simulink model "CM475A_TSG31CfgAndUse"  (R2013b)
settings: Solver=FixedStepDiscrete  SolverMode=SingleTasking  StartTime=0.0  StopTime=0.5  FixedStep=0.00005  RelTol=1e-3
undefined symbols (not defined in the file): ELECGLBPRM_PWMPERDMIN_NANOSEC_U32, sigbuilder_block, SysSt1, TSG31CfgAndUseAdcStrtOfCnvn2Offs, TSG31CfgAndUseAdcStrtOfCnvnMotCtrlPeakOffs, TSG31CfgAndUseAdcStrtOfCnvnMotCtrlVlyOffs, TSG31CfgAndUseMtrAg0SPIStart, TSG31CfgAndUsePwmDbnd, TSG31UPD_NANOSEC_U32
libraries: simulink x11, CM475A_TSG31CfgAndUse_ModelLibrary_Rev001 x11
(part 2 of 4)

== system CM475A_TSG31CfgAndUse/TSG31CfgAndUse/TSG31CfgAndUsePer2/No Transition SysState = Enable/MCECS_GAINCMDCF ==
  Action Port : ActionPort  ActionType=case
  CopyRight2 : Subsystem  Description=|  mask(Copyright Information){none=on}
      | Copyright info block.                                               
      |                                                                     
      | Place copyright information at the top of every subsystem in design.
      mask prompts: none "No parameters"
      mask help: Place copyright information at the top of every subsystem in design.
      mask Display:
      | NxtrConf = 'Nexteer Confidential';
      | 
      | sys = bdroot; %handle for the current model ("system")
      | first = get_param(sys,'Created');
      | first = first(end-3:end);  %year is last four digits
      | 
      | last = get_param(sys,'LastModifiedDate');
      | if isempty(last)
      |     last = datestr(now,'yyyy');
      | else
      |     last = last(end-3:end);
      | end
      | 
      | if strcmp(first,last)
      |     fprintf('%s -- Copyright %s Nexteer',NxtrConf,first)
      | else
      |     fprintf('%s -- %s%s- %s Nexteer',NxtrConf,char(169),first,last)
      | end
  Map Pins to GPIO : Subsystem  Priority=10  TreatAsAtomicUnit=on
      settings: AttributesFormatString=|
      | Priority:
      | %<Priority>
  Set GPIO Level : Subsystem  Priority=20  TreatAsAtomicUnit=on
      settings: AttributesFormatString=|
      | Priority:
      | %<Priority>

== system CM475A_TSG31CfgAndUse/TSG31CfgAndUse/TSG31CfgAndUsePer2/No Transition SysState = Enable/MCECS_OFFSCMDEND and MCECS_GAINCMDAD ==
  Action Port : ActionPort  ActionType=case
  CopyRight2 : Subsystem  Description=|  mask(Copyright Information){none=on}
      | Copyright info block.                                               
      |                                                                     
      | Place copyright information at the top of every subsystem in design.
      mask prompts: none "No parameters"
      mask help: Place copyright information at the top of every subsystem in design.
      mask Display:
      | NxtrConf = 'Nexteer Confidential';
      | 
      | sys = bdroot; %handle for the current model ("system")
      | first = get_param(sys,'Created');
      | first = first(end-3:end);  %year is last four digits
      | 
      | last = get_param(sys,'LastModifiedDate');
      | if isempty(last)
      |     last = datestr(now,'yyyy');
      | else
      |     last = last(end-3:end);
      | end
      | 
      | if strcmp(first,last)
      |     fprintf('%s -- Copyright %s Nexteer',NxtrConf,first)
      | else
      |     fprintf('%s -- %s%s- %s Nexteer',NxtrConf,char(169),first,last)
      | end
  Map Pins to GPIO : Subsystem  Priority=10  TreatAsAtomicUnit=on
      settings: AttributesFormatString=|
      | Priority:
      | %<Priority>
  Set GPIO Level : Subsystem  Priority=20  TreatAsAtomicUnit=on
      settings: AttributesFormatString=|
      | Priority:
      | %<Priority>

== system CM475A_TSG31CfgAndUse/TSG31CfgAndUse/TSG31CfgAndUsePer2/Transition from Enable/CopyRight2 ==

== system CM475A_TSG31CfgAndUse/TSG31CfgAndUse/TSG31CfgAndUsePer2/Transition from Enable/Map FET Ctrl Signals to GPIO and Set Low ==
  CopyRight2 : Subsystem  Description=|  mask(Copyright Information){none=on}
      | Copyright info block.                                               
      |                                                                     
      | Place copyright information at the top of every subsystem in design.
      mask prompts: none "No parameters"
      mask help: Place copyright information at the top of every subsystem in design.
      mask Display:
      | NxtrConf = 'Nexteer Confidential';
      | 
      | sys = bdroot; %handle for the current model ("system")
      | first = get_param(sys,'Created');
      | first = first(end-3:end);  %year is last four digits
      | 
      | last = get_param(sys,'LastModifiedDate');
      | if isempty(last)
      |     last = datestr(now,'yyyy');
      | else
      |     last = last(end-3:end);
      | end
      | 
      | if strcmp(first,last)
      |     fprintf('%s -- Copyright %s Nexteer',NxtrConf,first)
      | else
      |     fprintf('%s -- %s%s- %s Nexteer',NxtrConf,char(169),first,last)
      | end
  Map Pins to GPIO : Subsystem  RequirementInfo={'linktype_rmi_doors' '000089b8 (/ESG Group/FDD Module Requirements/ES FDDs/CM475A - TSG31 Configuration and Use)' '#CM475A_15' 'true' 'REQ: CM475A_15' '' } %GIDa_06ec1fec_3e1a_4ad4_824a_b175bdae6a2a  Priority=10  TreatAsAtomicUnit=on
      settings: AttributesFormatString=|
      | Priority:
      | %<Priority>
  Set GPIO Level : Subsystem  Priority=20  TreatAsAtomicUnit=on
      settings: AttributesFormatString=|
      | Priority:
      | %<Priority>

== system CM475A_TSG31CfgAndUse/TSG31CfgAndUse/TSG31CfgAndUsePer2/Transition to Enable/CopyRight2 ==

== system CM475A_TSG31CfgAndUse/TSG31CfgAndUse/TSG31CfgAndUsePer2/Transition to Enable/Map Pins to Peripheral ==
  IoHwAb_SetFctPeriphPhaALowrCmd : Subsystem  TreatAsAtomicUnit=on
  IoHwAb_SetFctPeriphPhaAUpprCmd : Subsystem  TreatAsAtomicUnit=on
  IoHwAb_SetFctPeriphPhaBLowrCmd : Subsystem  TreatAsAtomicUnit=on
  IoHwAb_SetFctPeriphPhaBUpprCmd : Subsystem  TreatAsAtomicUnit=on
  IoHwAb_SetFctPeriphPhaCLowrCmd : Subsystem  TreatAsAtomicUnit=on
  IoHwAb_SetFctPeriphPhaCUpprCmd : Subsystem  TreatAsAtomicUnit=on

== system CM475A_TSG31CfgAndUse/TSG31CfgAndUse/TSG31CfgAndUseInit1/Map FET Ctrl Signals to GPIO and Set Low/Map Pins to GPIO/CopyRight2 ==

== system CM475A_TSG31CfgAndUse/TSG31CfgAndUse/TSG31CfgAndUseInit1/Map FET Ctrl Signals to GPIO and Set Low/Map Pins to GPIO/IoHwAb_SetFctGpioPhaALowrCmd ==
  CopyRight2 : Subsystem  Description=|  mask(Copyright Information){none=on}
      | Copyright info block.                                               
      |                                                                     
      | Place copyright information at the top of every subsystem in design.
      mask prompts: none "No parameters"
      mask help: Place copyright information at the top of every subsystem in design.
      mask Display:
      | NxtrConf = 'Nexteer Confidential';
      | 
      | sys = bdroot; %handle for the current model ("system")
      | first = get_param(sys,'Created');
      | first = first(end-3:end);  %year is last four digits
      | 
      | last = get_param(sys,'LastModifiedDate');
      | if isempty(last)
      |     last = datestr(now,'yyyy');
      | else
      |     last = last(end-3:end);
      | end
      | 
      | if strcmp(first,last)
      |     fprintf('%s -- Copyright %s Nexteer',NxtrConf,first)
      | else
      |     fprintf('%s -- %s%s- %s Nexteer',NxtrConf,char(169),first,last)
      | end

== system CM475A_TSG31CfgAndUse/TSG31CfgAndUse/TSG31CfgAndUseInit1/Map FET Ctrl Signals to GPIO and Set Low/Map Pins to GPIO/IoHwAb_SetFctGpioPhaAUpprCmd ==
  CopyRight2 : Subsystem  Description=|  mask(Copyright Information){none=on}
      | Copyright info block.                                               
      |                                                                     
      | Place copyright information at the top of every subsystem in design.
      mask prompts: none "No parameters"
      mask help: Place copyright information at the top of every subsystem in design.
      mask Display:
      | NxtrConf = 'Nexteer Confidential';
      | 
      | sys = bdroot; %handle for the current model ("system")
      | first = get_param(sys,'Created');
      | first = first(end-3:end);  %year is last four digits
      | 
      | last = get_param(sys,'LastModifiedDate');
      | if isempty(last)
      |     last = datestr(now,'yyyy');
      | else
      |     last = last(end-3:end);
      | end
      | 
      | if strcmp(first,last)
      |     fprintf('%s -- Copyright %s Nexteer',NxtrConf,first)
      | else
      |     fprintf('%s -- %s%s- %s Nexteer',NxtrConf,char(169),first,last)
      | end

== system CM475A_TSG31CfgAndUse/TSG31CfgAndUse/TSG31CfgAndUseInit1/Map FET Ctrl Signals to GPIO and Set Low/Map Pins to GPIO/IoHwAb_SetFctGpioPhaBLowrCmd ==
  CopyRight2 : Subsystem  Description=|  mask(Copyright Information){none=on}
      | Copyright info block.                                               
      |                                                                     
      | Place copyright information at the top of every subsystem in design.
      mask prompts: none "No parameters"
      mask help: Place copyright information at the top of every subsystem in design.
      mask Display:
      | NxtrConf = 'Nexteer Confidential';
      | 
      | sys = bdroot; %handle for the current model ("system")
      | first = get_param(sys,'Created');
      | first = first(end-3:end);  %year is last four digits
      | 
      | last = get_param(sys,'LastModifiedDate');
      | if isempty(last)
      |     last = datestr(now,'yyyy');
      | else
      |     last = last(end-3:end);
      | end
      | 
      | if strcmp(first,last)
      |     fprintf('%s -- Copyright %s Nexteer',NxtrConf,first)
      | else
      |     fprintf('%s -- %s%s- %s Nexteer',NxtrConf,char(169),first,last)
      | end

== system CM475A_TSG31CfgAndUse/TSG31CfgAndUse/TSG31CfgAndUseInit1/Map FET Ctrl Signals to GPIO and Set Low/Map Pins to GPIO/IoHwAb_SetFctGpioPhaBUpprCmd ==
  CopyRight2 : Subsystem  Description=|  mask(Copyright Information){none=on}
      | Copyright info block.                                               
      |                                                                     
      | Place copyright information at the top of every subsystem in design.
      mask prompts: none "No parameters"
      mask help: Place copyright information at the top of every subsystem in design.
      mask Display:
      | NxtrConf = 'Nexteer Confidential';
      | 
      | sys = bdroot; %handle for the current model ("system")
      | first = get_param(sys,'Created');
      | first = first(end-3:end);  %year is last four digits
      | 
      | last = get_param(sys,'LastModifiedDate');
      | if isempty(last)
      |     last = datestr(now,'yyyy');
      | else
      |     last = last(end-3:end);
      | end
      | 
      | if strcmp(first,last)
      |     fprintf('%s -- Copyright %s Nexteer',NxtrConf,first)
      | else
      |     fprintf('%s -- %s%s- %s Nexteer',NxtrConf,char(169),first,last)
      | end

== system CM475A_TSG31CfgAndUse/TSG31CfgAndUse/TSG31CfgAndUseInit1/Map FET Ctrl Signals to GPIO and Set Low/Map Pins to GPIO/IoHwAb_SetFctGpioPhaCLowrCmd ==
  CopyRight2 : Subsystem  Description=|  mask(Copyright Information){none=on}
      | Copyright info block.                                               
      |                                                                     
      | Place copyright information at the top of every subsystem in design.
      mask prompts: none "No parameters"
      mask help: Place copyright information at the top of every subsystem in design.
      mask Display:
      | NxtrConf = 'Nexteer Confidential';
      | 
      | sys = bdroot; %handle for the current model ("system")
      | first = get_param(sys,'Created');
      | first = first(end-3:end);  %year is last four digits
      | 
      | last = get_param(sys,'LastModifiedDate');
      | if isempty(last)
      |     last = datestr(now,'yyyy');
      | else
      |     last = last(end-3:end);
      | end
      | 
      | if strcmp(first,last)
      |     fprintf('%s -- Copyright %s Nexteer',NxtrConf,first)
      | else
      |     fprintf('%s -- %s%s- %s Nexteer',NxtrConf,char(169),first,last)
      | end

== system CM475A_TSG31CfgAndUse/TSG31CfgAndUse/TSG31CfgAndUseInit1/Map FET Ctrl Signals to GPIO and Set Low/Map Pins to GPIO/IoHwAb_SetFctGpioPhaCUpprCmd ==
  CopyRight2 : Subsystem  Description=|  mask(Copyright Information){none=on}
      | Copyright info block.                                               
      |                                                                     
      | Place copyright information at the top of every subsystem in design.
      mask prompts: none "No parameters"
      mask help: Place copyright information at the top of every subsystem in design.
      mask Display:
      | NxtrConf = 'Nexteer Confidential';
      | 
      | sys = bdroot; %handle for the current model ("system")
      | first = get_param(sys,'Created');
      | first = first(end-3:end);  %year is last four digits
      | 
      | last = get_param(sys,'LastModifiedDate');
      | if isempty(last)
      |     last = datestr(now,'yyyy');
      | else
      |     last = last(end-3:end);
      | end
      | 
      | if strcmp(first,last)
      |     fprintf('%s -- Copyright %s Nexteer',NxtrConf,first)
      | else
      |     fprintf('%s -- %s%s- %s Nexteer',NxtrConf,char(169),first,last)
      | end

== system CM475A_TSG31CfgAndUse/TSG31CfgAndUse/TSG31CfgAndUseInit1/Map FET Ctrl Signals to GPIO and Set Low/Set GPIO Level/CopyRight2 ==

== system CM475A_TSG31CfgAndUse/TSG31CfgAndUse/TSG31CfgAndUseInit1/Map FET Ctrl Signals to GPIO and Set Low/Set GPIO Level/IoHwAb_SetGpioPhaALowrCmd ==
  PinSt : Inport  OutDataTypeStr=boolean
  CopyRight2 : Subsystem  Description=|  mask(Copyright Information){none=on}
      | Copyright info block.                                               
      |                                                                     
      | Place copyright information at the top of every subsystem in design.
      mask prompts: none "No parameters"
      mask help: Place copyright information at the top of every subsystem in design.
      mask Display:
      | NxtrConf = 'Nexteer Confidential';
      | 
      | sys = bdroot; %handle for the current model ("system")
      | first = get_param(sys,'Created');
      | first = first(end-3:end);  %year is last four digits
      | 
      | last = get_param(sys,'LastModifiedDate');
      | if isempty(last)
      |     last = datestr(now,'yyyy');
      | else
      |     last = last(end-3:end);
      | end
      | 
      | if strcmp(first,last)
      |     fprintf('%s -- Copyright %s Nexteer',NxtrConf,first)
      | else
      |     fprintf('%s -- %s%s- %s Nexteer',NxtrConf,char(169),first,last)
      | end
  Terminator : Terminator
  wires:
  PinSt/1 -> Terminator/1

== system CM475A_TSG31CfgAndUse/TSG31CfgAndUse/TSG31CfgAndUseInit1/Map FET Ctrl Signals to GPIO and Set Low/Set GPIO Level/IoHwAb_SetGpioPhaAUpprCmd ==
  PinSt : Inport  OutDataTypeStr=boolean
  CopyRight2 : Subsystem  Description=|  mask(Copyright Information){none=on}
      | Copyright info block.                                               
      |                                                                     
      | Place copyright information at the top of every subsystem in design.
      mask prompts: none "No parameters"
      mask help: Place copyright information at the top of every subsystem in design.
      mask Display:
      | NxtrConf = 'Nexteer Confidential';
      | 
      | sys = bdroot; %handle for the current model ("system")
      | first = get_param(sys,'Created');
      | first = first(end-3:end);  %year is last four digits
      | 
      | last = get_param(sys,'LastModifiedDate');
      | if isempty(last)
      |     last = datestr(now,'yyyy');
      | else
      |     last = last(end-3:end);
      | end
      | 
      | if strcmp(first,last)
      |     fprintf('%s -- Copyright %s Nexteer',NxtrConf,first)
      | else
      |     fprintf('%s -- %s%s- %s Nexteer',NxtrConf,char(169),first,last)
      | end
  Terminator : Terminator
  wires:
  PinSt/1 -> Terminator/1

== system CM475A_TSG31CfgAndUse/TSG31CfgAndUse/TSG31CfgAndUseInit1/Map FET Ctrl Signals to GPIO and Set Low/Set GPIO Level/IoHwAb_SetGpioPhaBLowrCmd ==
  PinSt : Inport  OutDataTypeStr=boolean
  CopyRight2 : Subsystem  Description=|  mask(Copyright Information){none=on}
      | Copyright info block.                                               
      |                                                                     
      | Place copyright information at the top of every subsystem in design.
      mask prompts: none "No parameters"
      mask help: Place copyright information at the top of every subsystem in design.
      mask Display:
      | NxtrConf = 'Nexteer Confidential';
      | 
      | sys = bdroot; %handle for the current model ("system")
      | first = get_param(sys,'Created');
      | first = first(end-3:end);  %year is last four digits
      | 
      | last = get_param(sys,'LastModifiedDate');
      | if isempty(last)
      |     last = datestr(now,'yyyy');
      | else
      |     last = last(end-3:end);
      | end
      | 
      | if strcmp(first,last)
      |     fprintf('%s -- Copyright %s Nexteer',NxtrConf,first)
      | else
      |     fprintf('%s -- %s%s- %s Nexteer',NxtrConf,char(169),first,last)
      | end
  Terminator : Terminator
  wires:
  PinSt/1 -> Terminator/1

== system CM475A_TSG31CfgAndUse/TSG31CfgAndUse/TSG31CfgAndUseInit1/Map FET Ctrl Signals to GPIO and Set Low/Set GPIO Level/IoHwAb_SetGpioPhaBUpprCmd ==
  PinSt : Inport  OutDataTypeStr=boolean
  CopyRight2 : Subsystem  Description=|  mask(Copyright Information){none=on}
      | Copyright info block.                                               
      |                                                                     
      | Place copyright information at the top of every subsystem in design.
      mask prompts: none "No parameters"
      mask help: Place copyright information at the top of every subsystem in design.
      mask Display:
      | NxtrConf = 'Nexteer Confidential';
      | 
      | sys = bdroot; %handle for the current model ("system")
      | first = get_param(sys,'Created');
      | first = first(end-3:end);  %year is last four digits
      | 
      | last = get_param(sys,'LastModifiedDate');
      | if isempty(last)
      |     last = datestr(now,'yyyy');
      | else
      |     last = last(end-3:end);
      | end
      | 
      | if strcmp(first,last)
      |     fprintf('%s -- Copyright %s Nexteer',NxtrConf,first)
      | else
      |     fprintf('%s -- %s%s- %s Nexteer',NxtrConf,char(169),first,last)
      | end
  Terminator : Terminator
  wires:
  PinSt/1 -> Terminator/1

== system CM475A_TSG31CfgAndUse/TSG31CfgAndUse/TSG31CfgAndUseInit1/Map FET Ctrl Signals to GPIO and Set Low/Set GPIO Level/IoHwAb_SetGpioPhaCLowrCmd ==
  PinSt : Inport  OutDataTypeStr=boolean
  CopyRight2 : Subsystem  Description=|  mask(Copyright Information){none=on}
      | Copyright info block.                                               
      |                                                                     
      | Place copyright information at the top of every subsystem in design.
      mask prompts: none "No parameters"
      mask help: Place copyright information at the top of every subsystem in design.
      mask Display:
      | NxtrConf = 'Nexteer Confidential';
      | 
      | sys = bdroot; %handle for the current model ("system")
      | first = get_param(sys,'Created');
      | first = first(end-3:end);  %year is last four digits
      | 
      | last = get_param(sys,'LastModifiedDate');
      | if isempty(last)
      |     last = datestr(now,'yyyy');
      | else
      |     last = last(end-3:end);
      | end
      | 
      | if strcmp(first,last)
      |     fprintf('%s -- Copyright %s Nexteer',NxtrConf,first)
      | else
      |     fprintf('%s -- %s%s- %s Nexteer',NxtrConf,char(169),first,last)
      | end
  Terminator : Terminator
  wires:
  PinSt/1 -> Terminator/1

== system CM475A_TSG31CfgAndUse/TSG31CfgAndUse/TSG31CfgAndUseInit1/Map FET Ctrl Signals to GPIO and Set Low/Set GPIO Level/IoHwAb_SetGpioPhaCUpprCmd ==
  PinSt : Inport  OutDataTypeStr=boolean
  CopyRight2 : Subsystem  Description=|  mask(Copyright Information){none=on}
      | Copyright info block.                                               
      |                                                                     
      | Place copyright information at the top of every subsystem in design.
      mask prompts: none "No parameters"
      mask help: Place copyright information at the top of every subsystem in design.
      mask Display:
      | NxtrConf = 'Nexteer Confidential';
      | 
      | sys = bdroot; %handle for the current model ("system")
      | first = get_param(sys,'Created');
      | first = first(end-3:end);  %year is last four digits
      | 
      | last = get_param(sys,'LastModifiedDate');
      | if isempty(last)
      |     last = datestr(now,'yyyy');
      | else
      |     last = last(end-3:end);
      | end
      | 
      | if strcmp(first,last)
      |     fprintf('%s -- Copyright %s Nexteer',NxtrConf,first)
      | else
      |     fprintf('%s -- %s%s- %s Nexteer',NxtrConf,char(169),first,last)
      | end
  Terminator : Terminator
  wires:
  PinSt/1 -> Terminator/1

== system CM475A_TSG31CfgAndUse/TSG31CfgAndUse/TSG31CfgAndUsePer2/No Transition SysState = Enable/Do Nothing/CopyRight2 ==

== system CM475A_TSG31CfgAndUse/TSG31CfgAndUse/TSG31CfgAndUsePer2/No Transition SysState = Enable/MCECS_CMDSAFEST/CopyRight2 ==

== system CM475A_TSG31CfgAndUse/TSG31CfgAndUse/TSG31CfgAndUsePer2/No Transition SysState = Enable/MCECS_CMDSAFEST/Map Pins to GPIO ==
  CopyRight2 : Subsystem  Description=|  mask(Copyright Information){none=on}
      | Copyright info block.                                               
      |                                                                     
      | Place copyright information at the top of every subsystem in design.
      mask prompts: none "No parameters"
      mask help: Place copyright information at the top of every subsystem in design.
      mask Display:
      | NxtrConf = 'Nexteer Confidential';
      | 
      | sys = bdroot; %handle for the current model ("system")
      | first = get_param(sys,'Created');
      | first = first(end-3:end);  %year is last four digits
      | 
      | last = get_param(sys,'LastModifiedDate');
      | if isempty(last)
      |     last = datestr(now,'yyyy');
      | else
      |     last = last(end-3:end);
      | end
      | 
      | if strcmp(first,last)
      |     fprintf('%s -- Copyright %s Nexteer',NxtrConf,first)
      | else
      |     fprintf('%s -- %s%s- %s Nexteer',NxtrConf,char(169),first,last)
      | end
  IoHwAb_SetFctGpioPhaALowrCmd : Subsystem  TreatAsAtomicUnit=on
  IoHwAb_SetFctGpioPhaAUpprCmd : Subsystem  TreatAsAtomicUnit=on
  IoHwAb_SetFctGpioPhaBLowrCmd : Subsystem  TreatAsAtomicUnit=on
  IoHwAb_SetFctGpioPhaBUpprCmd : Subsystem  TreatAsAtomicUnit=on
  IoHwAb_SetFctGpioPhaCLowrCmd : Subsystem  TreatAsAtomicUnit=on
  IoHwAb_SetFctGpioPhaCUpprCmd : Subsystem  TreatAsAtomicUnit=on

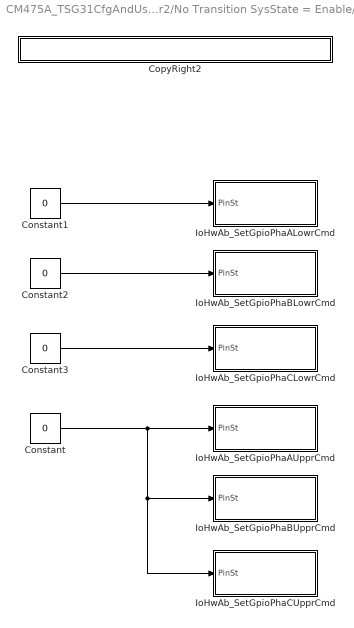
== system CM475A_TSG31CfgAndUse/TSG31CfgAndUse/TSG31CfgAndUsePer2/No Transition SysState = Enable/MCECS_CMDSAFEST/Set GPIO Level ==
  Constant{,1..3} (4 alike) : Constant  Value=0  OutDataTypeStr=boolean
  CopyRight2 : Subsystem  Description=|  mask(Copyright Information){none=on}
      | Copyright info block.                                               
      |                                                                     
      | Place copyright information at the top of every subsystem in design.
      mask prompts: none "No parameters"
      mask help: Place copyright information at the top of every subsystem in design.
      mask Display:
      | NxtrConf = 'Nexteer Confidential';
      | 
      | sys = bdroot; %handle for the current model ("system")
      | first = get_param(sys,'Created');
      | first = first(end-3:end);  %year is last four digits
      | 
      | last = get_param(sys,'LastModifiedDate');
      | if isempty(last)
      |     last = datestr(now,'yyyy');
      | else
      |     last = last(end-3:end);
      | end
      | 
      | if strcmp(first,last)
      |     fprintf('%s -- Copyright %s Nexteer',NxtrConf,first)
      | else
      |     fprintf('%s -- %s%s- %s Nexteer',NxtrConf,char(169),first,last)
      | end
  IoHwAb_SetGpioPhaALowrCmd : Subsystem  TreatAsAtomicUnit=on
  IoHwAb_SetGpioPhaAUpprCmd : Subsystem  TreatAsAtomicUnit=on
  IoHwAb_SetGpioPhaBLowrCmd : Subsystem  TreatAsAtomicUnit=on
  IoHwAb_SetGpioPhaBUpprCmd : Subsystem  TreatAsAtomicUnit=on
  IoHwAb_SetGpioPhaCLowrCmd : Subsystem  TreatAsAtomicUnit=on
  IoHwAb_SetGpioPhaCUpprCmd : Subsystem  TreatAsAtomicUnit=on
  wires:
  Constant3/1 -> IoHwAb_SetGpioPhaCLowrCmd/1(PinSt)
  Constant2/1 -> IoHwAb_SetGpioPhaBLowrCmd/1(PinSt)
  Constant1/1 -> IoHwAb_SetGpioPhaALowrCmd/1(PinSt)
  Constant/1 -> IoHwAb_SetGpioPhaAUpprCmd/1(PinSt), IoHwAb_SetGpioPhaBUpprCmd/1(PinSt), IoHwAb_SetGpioPhaCUpprCmd/1(PinSt)

== system CM475A_TSG31CfgAndUse/TSG31CfgAndUse/TSG31CfgAndUsePer2/No Transition SysState = Enable/MCECS_GAINCMDBE/CopyRight2 ==

== system CM475A_TSG31CfgAndUse/TSG31CfgAndUse/TSG31CfgAndUsePer2/No Transition SysState = Enable/MCECS_GAINCMDBE/Map Pins to GPIO ==
  CopyRight2 : Subsystem  Description=|  mask(Copyright Information){none=on}
      | Copyright info block.                                               
      |                                                                     
      | Place copyright information at the top of every subsystem in design.
      mask prompts: none "No parameters"
      mask help: Place copyright information at the top of every subsystem in design.
      mask Display:
      | NxtrConf = 'Nexteer Confidential';
      | 
      | sys = bdroot; %handle for the current model ("system")
      | first = get_param(sys,'Created');
      | first = first(end-3:end);  %year is last four digits
      | 
      | last = get_param(sys,'LastModifiedDate');
      | if isempty(last)
      |     last = datestr(now,'yyyy');
      | else
      |     last = last(end-3:end);
      | end
      | 
      | if strcmp(first,last)
      |     fprintf('%s -- Copyright %s Nexteer',NxtrConf,first)
      | else
      |     fprintf('%s -- %s%s- %s Nexteer',NxtrConf,char(169),first,last)
      | end
  IoHwAb_SetFctGpioPhaALowrCmd : Subsystem  TreatAsAtomicUnit=on
  IoHwAb_SetFctGpioPhaAUpprCmd : Subsystem  TreatAsAtomicUnit=on
  IoHwAb_SetFctGpioPhaBLowrCmd : Subsystem  TreatAsAtomicUnit=on
  IoHwAb_SetFctGpioPhaBUpprCmd : Subsystem  TreatAsAtomicUnit=on
  IoHwAb_SetFctGpioPhaCLowrCmd : Subsystem  TreatAsAtomicUnit=on
  IoHwAb_SetFctGpioPhaCUpprCmd : Subsystem  TreatAsAtomicUnit=on

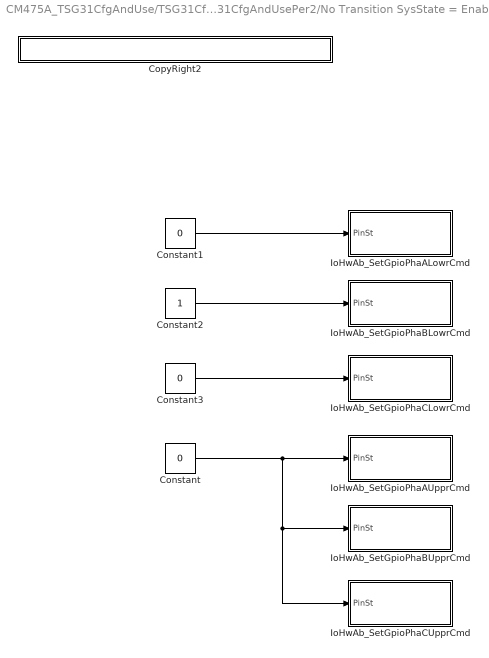
== system CM475A_TSG31CfgAndUse/TSG31CfgAndUse/TSG31CfgAndUsePer2/No Transition SysState = Enable/MCECS_GAINCMDBE/Set GPIO Level ==
  Constant : Constant  Value=0  OutDataTypeStr=boolean
  Constant1 : Constant  Value=0  OutDataTypeStr=boolean
  Constant2 : Constant  OutDataTypeStr=boolean
  Constant3 : Constant  Value=0  OutDataTypeStr=boolean
  CopyRight2 : Subsystem  Description=|  mask(Copyright Information){none=on}
      | Copyright info block.                                               
      |                                                                     
      | Place copyright information at the top of every subsystem in design.
      mask prompts: none "No parameters"
      mask help: Place copyright information at the top of every subsystem in design.
      mask Display:
      | NxtrConf = 'Nexteer Confidential';
      | 
      | sys = bdroot; %handle for the current model ("system")
      | first = get_param(sys,'Created');
      | first = first(end-3:end);  %year is last four digits
      | 
      | last = get_param(sys,'LastModifiedDate');
      | if isempty(last)
      |     last = datestr(now,'yyyy');
      | else
      |     last = last(end-3:end);
      | end
      | 
      | if strcmp(first,last)
      |     fprintf('%s -- Copyright %s Nexteer',NxtrConf,first)
      | else
      |     fprintf('%s -- %s%s- %s Nexteer',NxtrConf,char(169),first,last)
      | end
  IoHwAb_SetGpioPhaALowrCmd : Subsystem  TreatAsAtomicUnit=on
  IoHwAb_SetGpioPhaAUpprCmd : Subsystem  TreatAsAtomicUnit=on
  IoHwAb_SetGpioPhaBLowrCmd : Subsystem  TreatAsAtomicUnit=on
  IoHwAb_SetGpioPhaBUpprCmd : Subsystem  TreatAsAtomicUnit=on
  IoHwAb_SetGpioPhaCLowrCmd : Subsystem  TreatAsAtomicUnit=on
  IoHwAb_SetGpioPhaCUpprCmd : Subsystem  TreatAsAtomicUnit=on
  wires:
  Constant3/1 -> IoHwAb_SetGpioPhaCLowrCmd/1(PinSt)
  Constant2/1 -> IoHwAb_SetGpioPhaBLowrCmd/1(PinSt)
  Constant1/1 -> IoHwAb_SetGpioPhaALowrCmd/1(PinSt)
  Constant/1 -> IoHwAb_SetGpioPhaAUpprCmd/1(PinSt), IoHwAb_SetGpioPhaBUpprCmd/1(PinSt), IoHwAb_SetGpioPhaCUpprCmd/1(PinSt)

== system CM475A_TSG31CfgAndUse/TSG31CfgAndUse/TSG31CfgAndUsePer2/No Transition SysState = Enable/MCECS_GAINCMDCF/CopyRight2 ==

== system CM475A_TSG31CfgAndUse/TSG31CfgAndUse/TSG31CfgAndUsePer2/No Transition SysState = Enable/MCECS_GAINCMDCF/Map Pins to GPIO ==
  CopyRight2 : Subsystem  Description=|  mask(Copyright Information){none=on}
      | Copyright info block.                                               
      |                                                                     
      | Place copyright information at the top of every subsystem in design.
      mask prompts: none "No parameters"
      mask help: Place copyright information at the top of every subsystem in design.
      mask Display:
      | NxtrConf = 'Nexteer Confidential';
      | 
      | sys = bdroot; %handle for the current model ("system")
      | first = get_param(sys,'Created');
      | first = first(end-3:end);  %year is last four digits
      | 
      | last = get_param(sys,'LastModifiedDate');
      | if isempty(last)
      |     last = datestr(now,'yyyy');
      | else
      |     last = last(end-3:end);
      | end
      | 
      | if strcmp(first,last)
      |     fprintf('%s -- Copyright %s Nexteer',NxtrConf,first)
      | else
      |     fprintf('%s -- %s%s- %s Nexteer',NxtrConf,char(169),first,last)
      | end
  IoHwAb_SetFctGpioPhaALowrCmd : Subsystem  TreatAsAtomicUnit=on
  IoHwAb_SetFctGpioPhaAUpprCmd : Subsystem  TreatAsAtomicUnit=on
  IoHwAb_SetFctGpioPhaBLowrCmd : Subsystem  TreatAsAtomicUnit=on
  IoHwAb_SetFctGpioPhaBUpprCmd : Subsystem  TreatAsAtomicUnit=on
  IoHwAb_SetFctGpioPhaCLowrCmd : Subsystem  TreatAsAtomicUnit=on
  IoHwAb_SetFctGpioPhaCUpprCmd : Subsystem  TreatAsAtomicUnit=on

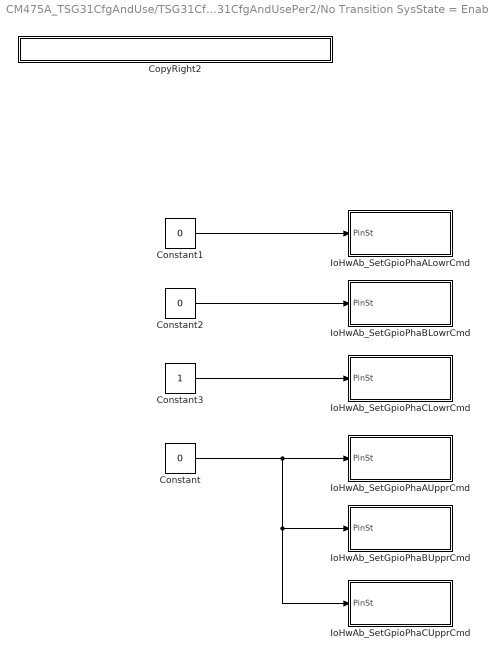
== system CM475A_TSG31CfgAndUse/TSG31CfgAndUse/TSG31CfgAndUsePer2/No Transition SysState = Enable/MCECS_GAINCMDCF/Set GPIO Level ==
  Constant : Constant  Value=0  OutDataTypeStr=boolean
  Constant1 : Constant  Value=0  OutDataTypeStr=boolean
  Constant2 : Constant  Value=0  OutDataTypeStr=boolean
  Constant3 : Constant  OutDataTypeStr=boolean
  CopyRight2 : Subsystem  Description=|  mask(Copyright Information){none=on}
      | Copyright info block.                                               
      |                                                                     
      | Place copyright information at the top of every subsystem in design.
      mask prompts: none "No parameters"
      mask help: Place copyright information at the top of every subsystem in design.
      mask Display:
      | NxtrConf = 'Nexteer Confidential';
      | 
      | sys = bdroot; %handle for the current model ("system")
      | first = get_param(sys,'Created');
      | first = first(end-3:end);  %year is last four digits
      | 
      | last = get_param(sys,'LastModifiedDate');
      | if isempty(last)
      |     last = datestr(now,'yyyy');
      | else
      |     last = last(end-3:end);
      | end
      | 
      | if strcmp(first,last)
      |     fprintf('%s -- Copyright %s Nexteer',NxtrConf,first)
      | else
      |     fprintf('%s -- %s%s- %s Nexteer',NxtrConf,char(169),first,last)
      | end
  IoHwAb_SetGpioPhaALowrCmd : Subsystem  TreatAsAtomicUnit=on
  IoHwAb_SetGpioPhaAUpprCmd : Subsystem  TreatAsAtomicUnit=on
  IoHwAb_SetGpioPhaBLowrCmd : Subsystem  TreatAsAtomicUnit=on
  IoHwAb_SetGpioPhaBUpprCmd : Subsystem  TreatAsAtomicUnit=on
  IoHwAb_SetGpioPhaCLowrCmd : Subsystem  TreatAsAtomicUnit=on
  IoHwAb_SetGpioPhaCUpprCmd : Subsystem  TreatAsAtomicUnit=on
  wires:
  Constant3/1 -> IoHwAb_SetGpioPhaCLowrCmd/1(PinSt)
  Constant2/1 -> IoHwAb_SetGpioPhaBLowrCmd/1(PinSt)
  Constant1/1 -> IoHwAb_SetGpioPhaALowrCmd/1(PinSt)
  Constant/1 -> IoHwAb_SetGpioPhaAUpprCmd/1(PinSt), IoHwAb_SetGpioPhaBUpprCmd/1(PinSt), IoHwAb_SetGpioPhaCUpprCmd/1(PinSt)

== system CM475A_TSG31CfgAndUse/TSG31CfgAndUse/TSG31CfgAndUsePer2/No Transition SysState = Enable/MCECS_OFFSCMDEND and MCECS_GAINCMDAD/CopyRight2 ==

== system CM475A_TSG31CfgAndUse/TSG31CfgAndUse/TSG31CfgAndUsePer2/No Transition SysState = Enable/MCECS_OFFSCMDEND and MCECS_GAINCMDAD/Map Pins to GPIO ==
  CopyRight2 : Subsystem  Description=|  mask(Copyright Information){none=on}
      | Copyright info block.                                               
      |                                                                     
      | Place copyright information at the top of every subsystem in design.
      mask prompts: none "No parameters"
      mask help: Place copyright information at the top of every subsystem in design.
      mask Display:
      | NxtrConf = 'Nexteer Confidential';
      | 
      | sys = bdroot; %handle for the current model ("system")
      | first = get_param(sys,'Created');
      | first = first(end-3:end);  %year is last four digits
      | 
      | last = get_param(sys,'LastModifiedDate');
      | if isempty(last)
      |     last = datestr(now,'yyyy');
      | else
      |     last = last(end-3:end);
      | end
      | 
      | if strcmp(first,last)
      |     fprintf('%s -- Copyright %s Nexteer',NxtrConf,first)
      | else
      |     fprintf('%s -- %s%s- %s Nexteer',NxtrConf,char(169),first,last)
      | end
  IoHwAb_SetFctGpioPhaALowrCmd : Subsystem  TreatAsAtomicUnit=on
  IoHwAb_SetFctGpioPhaAUpprCmd : Subsystem  TreatAsAtomicUnit=on
  IoHwAb_SetFctGpioPhaBLowrCmd : Subsystem  TreatAsAtomicUnit=on
  IoHwAb_SetFctGpioPhaBUpprCmd : Subsystem  TreatAsAtomicUnit=on
  IoHwAb_SetFctGpioPhaCLowrCmd : Subsystem  TreatAsAtomicUnit=on
  IoHwAb_SetFctGpioPhaCUpprCmd : Subsystem  TreatAsAtomicUnit=on

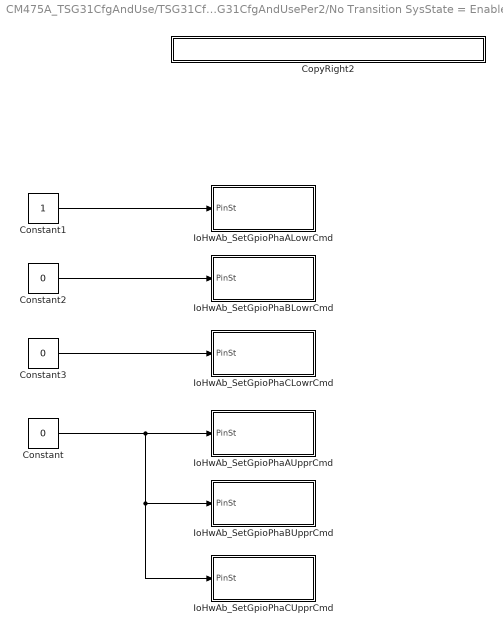
== system CM475A_TSG31CfgAndUse/TSG31CfgAndUse/TSG31CfgAndUsePer2/No Transition SysState = Enable/MCECS_OFFSCMDEND and MCECS_GAINCMDAD/Set GPIO Level ==
  Constant : Constant  Value=0  OutDataTypeStr=boolean
  Constant1 : Constant  OutDataTypeStr=boolean
  Constant2 : Constant  Value=0  OutDataTypeStr=boolean
  Constant3 : Constant  Value=0  OutDataTypeStr=boolean
  CopyRight2 : Subsystem  Description=|  mask(Copyright Information){none=on}
      | Copyright info block.                                               
      |                                                                     
      | Place copyright information at the top of every subsystem in design.
      mask prompts: none "No parameters"
      mask help: Place copyright information at the top of every subsystem in design.
      mask Display:
      | NxtrConf = 'Nexteer Confidential';
      | 
      | sys = bdroot; %handle for the current model ("system")
      | first = get_param(sys,'Created');
      | first = first(end-3:end);  %year is last four digits
      | 
      | last = get_param(sys,'LastModifiedDate');
      | if isempty(last)
      |     last = datestr(now,'yyyy');
      | else
      |     last = last(end-3:end);
      | end
      | 
      | if strcmp(first,last)
      |     fprintf('%s -- Copyright %s Nexteer',NxtrConf,first)
      | else
      |     fprintf('%s -- %s%s- %s Nexteer',NxtrConf,char(169),first,last)
      | end
  IoHwAb_SetGpioPhaALowrCmd : Subsystem  TreatAsAtomicUnit=on
  IoHwAb_SetGpioPhaAUpprCmd : Subsystem  TreatAsAtomicUnit=on
  IoHwAb_SetGpioPhaBLowrCmd : Subsystem  TreatAsAtomicUnit=on
  IoHwAb_SetGpioPhaBUpprCmd : Subsystem  TreatAsAtomicUnit=on
  IoHwAb_SetGpioPhaCLowrCmd : Subsystem  TreatAsAtomicUnit=on
  IoHwAb_SetGpioPhaCUpprCmd : Subsystem  TreatAsAtomicUnit=on
  wires:
  Constant/1 -> IoHwAb_SetGpioPhaCUpprCmd/1(PinSt), IoHwAb_SetGpioPhaBUpprCmd/1(PinSt), IoHwAb_SetGpioPhaAUpprCmd/1(PinSt)
  Constant1/1 -> IoHwAb_SetGpioPhaALowrCmd/1(PinSt)
  Constant2/1 -> IoHwAb_SetGpioPhaBLowrCmd/1(PinSt)
  Constant3/1 -> IoHwAb_SetGpioPhaCLowrCmd/1(PinSt)

== system CM475A_TSG31CfgAndUse/TSG31CfgAndUse/TSG31CfgAndUsePer2/Transition from Enable/Map FET Ctrl Signals to GPIO and Set Low/CopyRight2 ==

== matlab function CM475A_TSG31CfgAndUse/TSG31CfgAndUse/TSG31CfgAndUsePer1/Truth Table ==
  data: MotCurrEolCalSt input uint8; PwmPeriod output uint32; PwmPerd input uint32; PhaOnTiA input uint32; PhaOnTiB input uint32; PhaOnTiC input uint32; PhaseAOnTime output uint32; PhaseBOnTime output uint32; PhaseCOnTime output uint32; CurrMeasEolOffsHiCmuOffs constant uint32; CurrMeasEolFixdPwmPerd constant uint32; CurrMeasEolOffsLoCmuOffs constant double
function [PwmPeriod, PhaseAOnTime, PhaseBOnTime, PhaseCOnTime] = fcn(MotCurrEolCalSt, PwmPerd, PhaOnTiA, PhaOnTiB, PhaOnTiC)

aVarTruthTableCondition_1 = false;
aVarTruthTableCondition_2 = false;
aVarTruthTableCondition_3 = false;
aVarTruthTableCondition_4 = false;


% Normal Operation
% MCECS_OFFSCMDSTRT (0)

aVarTruthTableCondition_1 = logical(MotCurrEolCalSt == 0);

% MCECS_OFFSCMDHI   (1)

aVarTruthTableCondition_2 = logical(MotCurrEolCalSt == 1);

% MCECS_OFFSCMDLO   (2)

aVarTruthTableCondition_3 = logical(MotCurrEolCalSt == 2);

% MCECS_OFFSCMDZERO (3)

aVarTruthTableCondition_4 = logical(MotCurrEolCalSt == 3);

if (aVarTruthTableCondition_2)
    aFcnTruthTableAction_1();
elseif (aVarTruthTableCondition_3)
    aFcnTruthTableAction_2();
elseif (aVarTruthTableCondition_4)
    aFcnTruthTableAction_3();
elseif (aVarTruthTableCondition_1)
    aFcnTruthTableAction_4();
else % Default
    aFcnTruthTableAction_4();
end

function aFcnTruthTableAction_1()

% MCECS_OFFSCMDHI   (1)

PwmPeriod = uint32(CurrMeasEolFixdPwmPerd);
PhaseAOnTime = uint32(CurrMeasEolOffsHiCmuOffs);
PhaseBOnTime = uint32(CurrMeasEolOffsHiCmuOffs);
PhaseCOnTime = uint32(CurrMeasEolOffsHiCmuOffs);

function aFcnTruthTableAction_2()

% MCECS_OFFSCMDLO   (2)

PwmPeriod = uint32(CurrMeasEolFixdPwmPerd);
PhaseAOnTime = uint32(CurrMeasEolOffsLoCmuOffs);
PhaseBOnTime = uint32(CurrMeasEolOffsLoCmuOffs);
PhaseCOnTime = uint32(CurrMeasEolOffsLoCmuOffs);

function aFcnTruthTableAction_3()

% MCECS_OFFSCMDZERO (3)

PwmPeriod = uint32(CurrMeasEolFixdPwmPerd);
PhaseAOnTime = uint32(0);
PhaseBOnTime = uint32(0);
PhaseCOnTime = uint32(0);

function aFcnTruthTableAction_4()

% Default

PwmPeriod = uint32(PwmPerd);
PhaseAOnTime = uint32(PhaOnTiA);
PhaseBOnTime = uint32(PhaOnTiB);
PhaseCOnTime = uint32(PhaOnTiC);

== system CM475A_TSG31CfgAndUse/TSG31CfgAndUse/TSG31CfgAndUsePer2/Transition from Enable/Map FET Ctrl Signals to GPIO and Set Low/Map Pins to GPIO ==
  CopyRight2 : Subsystem  Description=|  mask(Copyright Information){none=on}
      | Copyright info block.                                               
      |                                                                     
      | Place copyright information at the top of every subsystem in design.
      mask prompts: none "No parameters"
      mask help: Place copyright information at the top of every subsystem in design.
      mask Display:
      | NxtrConf = 'Nexteer Confidential';
      | 
      | sys = bdroot; %handle for the current model ("system")
      | first = get_param(sys,'Created');
      | first = first(end-3:end);  %year is last four digits
      | 
      | last = get_param(sys,'LastModifiedDate');
      | if isempty(last)
      |     last = datestr(now,'yyyy');
      | else
      |     last = last(end-3:end);
      | end
      | 
      | if strcmp(first,last)
      |     fprintf('%s -- Copyright %s Nexteer',NxtrConf,first)
      | else
      |     fprintf('%s -- %s%s- %s Nexteer',NxtrConf,char(169),first,last)
      | end
  IoHwAb_SetFctGpioPhaALowrCmd : Subsystem  TreatAsAtomicUnit=on
  IoHwAb_SetFctGpioPhaAUpprCmd : Subsystem  TreatAsAtomicUnit=on
  IoHwAb_SetFctGpioPhaBLowrCmd : Subsystem  TreatAsAtomicUnit=on
  IoHwAb_SetFctGpioPhaBUpprCmd : Subsystem  TreatAsAtomicUnit=on
  IoHwAb_SetFctGpioPhaCLowrCmd : Subsystem  TreatAsAtomicUnit=on
  IoHwAb_SetFctGpioPhaCUpprCmd : Subsystem  TreatAsAtomicUnit=on

== system CM475A_TSG31CfgAndUse/TSG31CfgAndUse/TSG31CfgAndUsePer2/Transition from Enable/Map FET Ctrl Signals to GPIO and Set Low/Set GPIO Level ==
  Constant : Constant  Value=0  OutDataTypeStr=boolean
  CopyRight2 : Subsystem  Description=|  mask(Copyright Information){none=on}
      | Copyright info block.                                               
      |                                                                     
      | Place copyright information at the top of every subsystem in design.
      mask prompts: none "No parameters"
      mask help: Place copyright information at the top of every subsystem in design.
      mask Display:
      | NxtrConf = 'Nexteer Confidential';
      | 
      | sys = bdroot; %handle for the current model ("system")
      | first = get_param(sys,'Created');
      | first = first(end-3:end);  %year is last four digits
      | 
      | last = get_param(sys,'LastModifiedDate');
      | if isempty(last)
      |     last = datestr(now,'yyyy');
      | else
      |     last = last(end-3:end);
      | end
      | 
      | if strcmp(first,last)
      |     fprintf('%s -- Copyright %s Nexteer',NxtrConf,first)
      | else
      |     fprintf('%s -- %s%s- %s Nexteer',NxtrConf,char(169),first,last)
      | end
  IoHwAb_SetGpioPhaALowrCmd : Subsystem  TreatAsAtomicUnit=on
  IoHwAb_SetGpioPhaAUpprCmd : Subsystem  TreatAsAtomicUnit=on
  IoHwAb_SetGpioPhaBLowrCmd : Subsystem  TreatAsAtomicUnit=on
  IoHwAb_SetGpioPhaBUpprCmd : Subsystem  TreatAsAtomicUnit=on
  IoHwAb_SetGpioPhaCLowrCmd : Subsystem  TreatAsAtomicUnit=on
  IoHwAb_SetGpioPhaCUpprCmd : Subsystem  TreatAsAtomicUnit=on
  wires:
  Constant/1 -> IoHwAb_SetGpioPhaALowrCmd/1(PinSt), IoHwAb_SetGpioPhaCUpprCmd/1(PinSt), IoHwAb_SetGpioPhaBUpprCmd/1(PinSt), IoHwAb_SetGpioPhaAUpprCmd/1(PinSt), IoHwAb_SetGpioPhaCLowrCmd/1(PinSt), IoHwAb_SetGpioPhaBLowrCmd/1(PinSt)

== system CM475A_TSG31CfgAndUse/TSG31CfgAndUse/TSG31CfgAndUsePer2/Transition to Enable/Map Pins to Peripheral/IoHwAb_SetFctPeriphPhaALowrCmd ==
  CopyRight2 : Subsystem  Description=|  mask(Copyright Information){none=on}
      | Copyright info block.                                               
      |                                                                     
      | Place copyright information at the top of every subsystem in design.
      mask prompts: none "No parameters"
      mask help: Place copyright information at the top of every subsystem in design.
      mask Display:
      | NxtrConf = 'Nexteer Confidential';
      | 
      | sys = bdroot; %handle for the current model ("system")
      | first = get_param(sys,'Created');
      | first = first(end-3:end);  %year is last four digits
      | 
      | last = get_param(sys,'LastModifiedDate');
      | if isempty(last)
      |     last = datestr(now,'yyyy');
      | else
      |     last = last(end-3:end);
      | end
      | 
      | if strcmp(first,last)
      |     fprintf('%s -- Copyright %s Nexteer',NxtrConf,first)
      | else
      |     fprintf('%s -- %s%s- %s Nexteer',NxtrConf,char(169),first,last)
      | end

== system CM475A_TSG31CfgAndUse/TSG31CfgAndUse/TSG31CfgAndUsePer2/Transition to Enable/Map Pins to Peripheral/IoHwAb_SetFctPeriphPhaAUpprCmd ==
  CopyRight2 : Subsystem  Description=|  mask(Copyright Information){none=on}
      | Copyright info block.                                               
      |                                                                     
      | Place copyright information at the top of every subsystem in design.
      mask prompts: none "No parameters"
      mask help: Place copyright information at the top of every subsystem in design.
      mask Display:
      | NxtrConf = 'Nexteer Confidential';
      | 
      | sys = bdroot; %handle for the current model ("system")
      | first = get_param(sys,'Created');
      | first = first(end-3:end);  %year is last four digits
      | 
      | last = get_param(sys,'LastModifiedDate');
      | if isempty(last)
      |     last = datestr(now,'yyyy');
      | else
      |     last = last(end-3:end);
      | end
      | 
      | if strcmp(first,last)
      |     fprintf('%s -- Copyright %s Nexteer',NxtrConf,first)
      | else
      |     fprintf('%s -- %s%s- %s Nexteer',NxtrConf,char(169),first,last)
      | end

== system CM475A_TSG31CfgAndUse/TSG31CfgAndUse/TSG31CfgAndUsePer2/Transition to Enable/Map Pins to Peripheral/IoHwAb_SetFctPeriphPhaBLowrCmd ==
  CopyRight2 : Subsystem  Description=|  mask(Copyright Information){none=on}
      | Copyright info block.                                               
      |                                                                     
      | Place copyright information at the top of every subsystem in design.
      mask prompts: none "No parameters"
      mask help: Place copyright information at the top of every subsystem in design.
      mask Display:
      | NxtrConf = 'Nexteer Confidential';
      | 
      | sys = bdroot; %handle for the current model ("system")
      | first = get_param(sys,'Created');
      | first = first(end-3:end);  %year is last four digits
      | 
      | last = get_param(sys,'LastModifiedDate');
      | if isempty(last)
      |     last = datestr(now,'yyyy');
      | else
      |     last = last(end-3:end);
      | end
      | 
      | if strcmp(first,last)
      |     fprintf('%s -- Copyright %s Nexteer',NxtrConf,first)
      | else
      |     fprintf('%s -- %s%s- %s Nexteer',NxtrConf,char(169),first,last)
      | end

== system CM475A_TSG31CfgAndUse/TSG31CfgAndUse/TSG31CfgAndUsePer2/Transition to Enable/Map Pins to Peripheral/IoHwAb_SetFctPeriphPhaBUpprCmd ==
  CopyRight2 : Subsystem  Description=|  mask(Copyright Information){none=on}
      | Copyright info block.                                               
      |                                                                     
      | Place copyright information at the top of every subsystem in design.
      mask prompts: none "No parameters"
      mask help: Place copyright information at the top of every subsystem in design.
      mask Display:
      | NxtrConf = 'Nexteer Confidential';
      | 
      | sys = bdroot; %handle for the current model ("system")
      | first = get_param(sys,'Created');
      | first = first(end-3:end);  %year is last four digits
      | 
      | last = get_param(sys,'LastModifiedDate');
      | if isempty(last)
      |     last = datestr(now,'yyyy');
      | else
      |     last = last(end-3:end);
      | end
      | 
      | if strcmp(first,last)
      |     fprintf('%s -- Copyright %s Nexteer',NxtrConf,first)
      | else
      |     fprintf('%s -- %s%s- %s Nexteer',NxtrConf,char(169),first,last)
      | end

== system CM475A_TSG31CfgAndUse/TSG31CfgAndUse/TSG31CfgAndUsePer2/Transition to Enable/Map Pins to Peripheral/IoHwAb_SetFctPeriphPhaCLowrCmd ==
  CopyRight2 : Subsystem  Description=|  mask(Copyright Information){none=on}
      | Copyright info block.                                               
      |                                                                     
      | Place copyright information at the top of every subsystem in design.
      mask prompts: none "No parameters"
      mask help: Place copyright information at the top of every subsystem in design.
      mask Display:
      | NxtrConf = 'Nexteer Confidential';
      | 
      | sys = bdroot; %handle for the current model ("system")
      | first = get_param(sys,'Created');
      | first = first(end-3:end);  %year is last four digits
      | 
      | last = get_param(sys,'LastModifiedDate');
      | if isempty(last)
      |     last = datestr(now,'yyyy');
      | else
      |     last = last(end-3:end);
      | end
      | 
      | if strcmp(first,last)
      |     fprintf('%s -- Copyright %s Nexteer',NxtrConf,first)
      | else
      |     fprintf('%s -- %s%s- %s Nexteer',NxtrConf,char(169),first,last)
      | end

== system CM475A_TSG31CfgAndUse/TSG31CfgAndUse/TSG31CfgAndUsePer2/Transition to Enable/Map Pins to Peripheral/IoHwAb_SetFctPeriphPhaCUpprCmd ==
  CopyRight2 : Subsystem  Description=|  mask(Copyright Information){none=on}
      | Copyright info block.                                               
      |                                                                     
      | Place copyright information at the top of every subsystem in design.
      mask prompts: none "No parameters"
      mask help: Place copyright information at the top of every subsystem in design.
      mask Display:
      | NxtrConf = 'Nexteer Confidential';
      | 
      | sys = bdroot; %handle for the current model ("system")
      | first = get_param(sys,'Created');
      | first = first(end-3:end);  %year is last four digits
      | 
      | last = get_param(sys,'LastModifiedDate');
      | if isempty(last)
      |     last = datestr(now,'yyyy');
      | else
      |     last = last(end-3:end);
      | end
      | 
      | if strcmp(first,last)
      |     fprintf('%s -- Copyright %s Nexteer',NxtrConf,first)
      | else
      |     fprintf('%s -- %s%s- %s Nexteer',NxtrConf,char(169),first,last)
      | end
